simulink model "qpRefinery"  (R2020a)
settings: Solver=VariableStepAuto  StartTime=0.0  StopTime=10.0  RelTol=1e-3
settings Model: Creator=eirik.engen  LastModifiedBy=eirik.engen

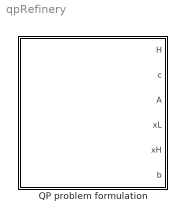
== system qpRefinery ==
  QP problem formulation : MATLAB Function  TreatAsAtomicUnit=on

== matlab function qpRefinery/QP problem formulation ==
  data: H output; c output; A output; xL output; xH output; b output
function [H,c,A,xL,xH,b] = QP_problem_refinery()

% make matrices and vectors

%Hessian matrix H
H_mat = diag([0,0,2/5000,2/5000,0,0]);

%qpOASES does not accept matrices, but only vectors
% whe have to change H matrix to vector by stacking elements column wise
H = H_mat(:);

%c matrix
%linear term vector
c=-[-24.5 -16 36 24 21 10];

%A matrix for linear equality constraints
%equality contstraints
A_mat = [0.80 0.44 -1 0 0 0
         0.05 0.10 0 -1 0 0
         0.10 0.36 0 0 -1 0
         0.05 0.10 0 0 0 -1];
A = A_mat(:);
